simulink model "Assignment2_group4"  (R2020a)
settings: Solver=FixedStepAuto  StartTime=0.0  StopTime=10.0  FixedStep=1e-3  RelTol=1e-3  EnableMultiTasking=on
undefined symbols (not defined in the file): A0, A1, D0, D1, D10, D11, D12, D13, D2, D3, D4, D5, D6, D7, D8, D9, PTA0, PTA1, PTA2, PTB2, PTB23, PTB3, PTB9, PTC16, PTC17, PTC2, PTC3, PTC4, PTD0, PTD1, PTD2, PTD3
libraries: frdmk64flib x23, etargetslib x2
settings Model: ExtModeTrigDuration=5  Creator=win10  LastModifiedBy=win10
settings OptimizationCC: EnhancedBackFolding=on  PassReuseOutputArgsAs=Individual arguments  ZeroExternalMemoryAtStartup=off  ZeroInternalMemoryAtStartup=off  MaxStackSize=64  OptimizeBlockOrder=speed  DifferentSizesBufferReuse=on  OptimizationCustomize=off  EfficientTunableParamExpr=on
settings DebuggingCC: ParameterTunabilityLossMsg=error
settings HardwareCC: ProdBitPerPointer=32  ProdBitPerSizeT=32  ProdBitPerPtrDiffT=32  ProdLargestAtomicInteger=Long  ProdLargestAtomicFloat=Double  ProdWordSize=32  ProdHWDeviceType=ARM Compatible->ARM Cortex
settings SFSimCC: MATLABDynamicMemAlloc=off
settings RTWCC: SystemTargetFile=ert.tlc  HardwareBoard=NXP FRDM-K64F  TemplateMakefile=ert_default_tmf  Toolchain=GNU Tools for ARM Embedded Processors
settings CodeAppCC: ForceParamTrailComments=on  IgnoreCustomStorageClasses=off  OperatorAnnotations=on  SimulinkDataObjDesc=on  SFDataObjDesc=on  InsertBlockDesc=on

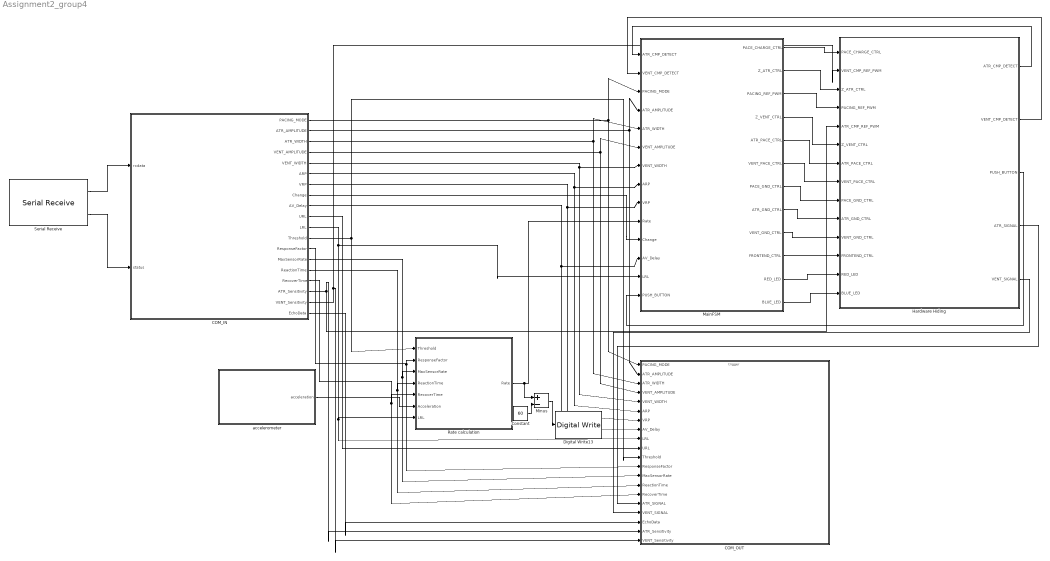
== system Assignment2_group4 ==
  COM_IN : Stateflow chart  TreatAsAtomicUnit=on
      settings: PortSchema="{\"entries\":[{\"content\":{\"sides\":[{\"content\":{\"connectorIds\":[\"In2\",\"In1\"]},\"type\":\"ConnectorPlacement.EquallySpacedRectSide\",\"uuid\":\"e3132103-f253-4432-b504-84705a150e61\"},{\"content\":{\"connectorIds\":[\"Out1\",\"Out2\",\"Out3\",\"Out4\",\"Out5\",\"Out6\",\"Out7\",\"Out8\",\"Out9\",\"Out10\",\"Out11\",\"Out12\",\"Out13\",\"Out14\",\"Out15\",\"Out16\",\"Out17\",\"Out18\",\"Out19\"],\"side\":\"RIGHT\"},\"type\":\"ConnectorPlacement.EquallySpacedRectSide\",\"uuid\":\"097bc9b8-1262-45b5-bb9b-69159a4df10c\"},{\"content\":{\"connectorIds\":[],\"side\":\"TOP\"},\"type\":\"ConnectorPlacement.EquallySpacedRectSide\",\"uuid\":\"fce19345-6d4b-4b3c-aee5-22ababb9e44d\"}]},\"type\":\"ConnectorPlacement.EquallySpacedConnector\",\"uuid\":\"5020afdc-7bbd-4924-8d59-6a0d5305ac11\"}],\"packageUris\":[\"http://schema.mathworks.com/mf0/Connector/19700101\"],\"version\":\"1.0\"}"
  COM_OUT : Subsystem  TreatAsAtomicUnit=on
  Constant : Constant  Value=60
  Digital Write13 : frdmk64flib/Digital Write  Whichpin=GREEN_LED
  Hardware Hiding : Subsystem
  MainFSM : Stateflow chart  TreatAsAtomicUnit=on
  Minus : Sum  Inputs=+-
  Rate calculation : Subsystem
  Serial Receive : frdmk64flib/Serial Receive  SCIModule=0  Baudrate=uint32(9600)  Parity=None  StopBits=1  HardwareFlowControl=None  ByteOrder=LittleEndian  DataType=uint8  DataLength=19  BlockingMode=off  OutputStatus=on  SampleTime=-1
  accelerometer : Subsystem
  wires:
  accelerometer/1(acceleration) -> Rate calculation/6(Acceleration)
  Rate calculation/1(Rate) -> Minus/1, MainFSM/10(Rate)
  Serial Receive/1 -> COM_IN/2(rxdata)
  Serial Receive/2 -> COM_IN/1(status)
  COM_IN/1(PACING_MODE) -> MainFSM/3(PACING_MODE), COM_OUT/1(PACING_MODE)
  COM_IN/5(VENT_WIDTH) -> COM_OUT/5(VENT_WIDTH), MainFSM/7(VENT_WIDTH)
  COM_IN/6(ARP) -> COM_OUT/6(ARP), MainFSM/8(ARP)
  COM_IN/7(VRP) -> COM_OUT/7(VRP), MainFSM/9(VRP)
  COM_IN/8(Change) -> MainFSM/11(Change)
  COM_IN/9(AV_Delay) -> COM_OUT/8(AV_Delay), MainFSM/12(AV_Delay)
  COM_IN/11(LRL) -> Rate calculation/7(LRL), COM_OUT/9(LRL), MainFSM/13(LRL)
  COM_IN/13(ResponseFactor) -> COM_OUT/12(ResponseFactor), Rate calculation/2(ResponseFactor)
  COM_IN/14(MaxSensorRate) -> COM_OUT/13(MaxSensorRate), Rate calculation/3(MaxSensorRate)
  COM_IN/15(ReactionTime) -> COM_OUT/14(ReactionTime), Rate calculation/4(ReactionTime)
  COM_IN/16(RecoverTime) -> Rate calculation/5(RecoverTime), COM_OUT/15(RecoverTime)
  COM_IN/10(URL) -> COM_OUT/10(URL)
  COM_IN/19(EchoData) -> COM_OUT/18(EchoData)
  COM_IN/3(ATR_WIDTH) -> MainFSM/5(ATR_WIDTH), COM_OUT/3(ATR_WIDTH)
  COM_IN/12(Threshold) -> COM_OUT/11(Threshold), Rate calculation/1(Threshold)
  COM_IN/4(VENT_AMPLITUDE) -> MainFSM/6(VENT_AMPLITUDE), COM_OUT/4(VENT_AMPLITUDE)
  COM_IN/2(ATR_AMPLITUDE) -> MainFSM/4(ATR_AMPLITUDE), COM_OUT/2(ATR_AMPLITUDE)
  COM_IN/17(ATR_Sensitivity) -> COM_OUT/19(ATR_Sensitivity), Hardware Hiding/5(ATR_CMP_REF_PWM)
  COM_IN/18(VENT_Sensitivity) -> Hardware Hiding/2(VENT_CMP_REF_PWM), COM_OUT/20(VENT_Sensitivity)
  MainFSM/1(PACE_CHARGE_CTRL) -> Hardware Hiding/1(PACE_CHARGE_CTRL)
  MainFSM/2(Z_ATR_CTRL) -> Hardware Hiding/3(Z_ATR_CTRL)
  MainFSM/3(PACING_REF_PWM) -> Hardware Hiding/4(PACING_REF_PWM)
  MainFSM/4(Z_VENT_CTRL) -> Hardware Hiding/6(Z_VENT_CTRL)
  MainFSM/5(ATR_PACE_CTRL) -> Hardware Hiding/7(ATR_PACE_CTRL)
  MainFSM/6(VENT_PACE_CTRL) -> Hardware Hiding/8(VENT_PACE_CTRL)
  MainFSM/7(PACE_GND_CTRL) -> Hardware Hiding/9(PACE_GND_CTRL)
  MainFSM/8(ATR_GND_CTRL) -> Hardware Hiding/10(ATR_GND_CTRL)
  MainFSM/9(VENT_GND_CTRL) -> Hardware Hiding/11(VENT_GND_CTRL)
  MainFSM/10(FRONTEND_CTRL) -> Hardware Hiding/12(FRONTEND_CTRL)
  MainFSM/11(RED_LED) -> Hardware Hiding/13(RED_LED)
  MainFSM/12(BLUE_LED) -> Hardware Hiding/14(BLUE_LED)
  Hardware Hiding/4(ATR_SIGNAL) -> COM_OUT/16(ATR_SIGNAL)
  Hardware Hiding/5(VENT_SIGNAL) -> COM_OUT/17(VENT_SIGNAL)
  Hardware Hiding/1(ATR_CMP_DETECT) -> MainFSM/1(ATR_CMP_DETECT)
  Hardware Hiding/2(VENT_CMP_DETECT) -> MainFSM/2(VENT_CMP_DETECT)
  Hardware Hiding/3(PUSH_BUTTON) -> MainFSM/14(PUSH_BUTTON)
  Constant/1 -> Minus/2
  Minus/1 -> Digital Write13/1

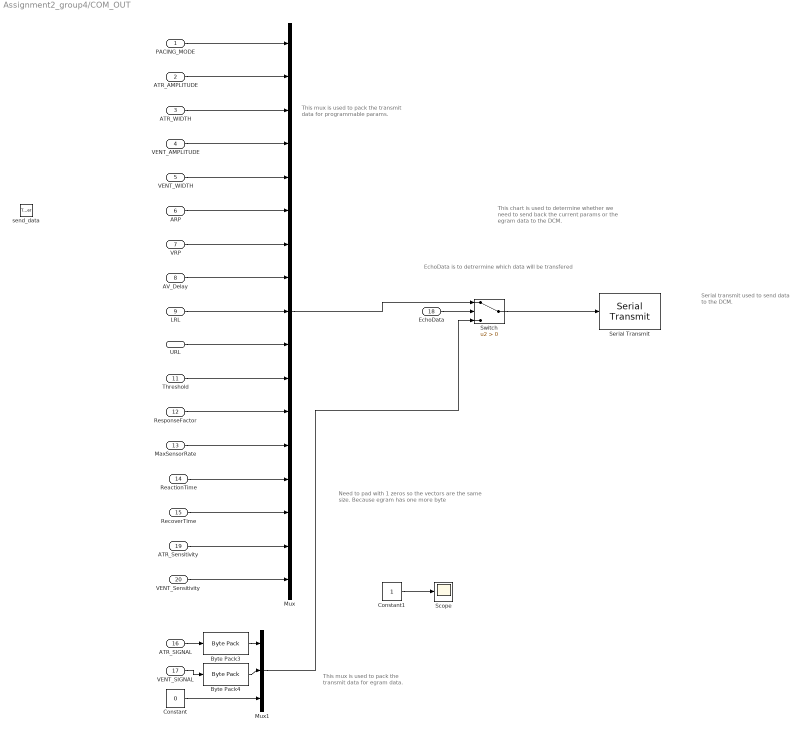
== system Assignment2_group4/COM_OUT ==
  note: EchoData is to detrermine which data will be transfered
  note: Serial transmit used to send data
      | to the DCM.
  note: This chart is used to determine whether
      | we need to send back the current params
      | or the egram data to the DCM.
  note: Need to pad with 1 zeros so the vectors
      | are the same size. Because egram has one more byte
  note: This mux is used to pack the
      | transmit data for egram data.
  note: This mux is used to pack the transmit
      | data for programmable params.
  PACING_MODE : Inport  OutDataTypeStr=uint8
  ATR_AMPLITUDE : Inport  Port=2  OutDataTypeStr=uint8
  ATR_WIDTH : Inport  Port=3  OutDataTypeStr=uint8
  VENT_AMPLITUDE : Inport  Port=4  OutDataTypeStr=uint8
  VENT_WIDTH : Inport  Port=5  OutDataTypeStr=uint8
  ARP : Inport  Port=6  OutDataTypeStr=uint8
  VRP : Inport  Port=7  OutDataTypeStr=uint8
  AV_Delay : Inport  Port=8  OutDataTypeStr=uint8
  LRL : Inport  Port=9  OutDataTypeStr=uint8
  URL : Inport  Port=10  OutDataTypeStr=uint8
  Threshold : Inport  Port=11  OutDataTypeStr=uint8
  ResponseFactor : Inport  Port=12  OutDataTypeStr=uint8
  MaxSensorRate : Inport  Port=13  OutDataTypeStr=uint8
  ReactionTime : Inport  Port=14  OutDataTypeStr=uint8
  RecoverTime : Inport  Port=15  OutDataTypeStr=uint8
  ATR_SIGNAL : Inport  Port=16  OutDataTypeStr=double
  VENT_SIGNAL : Inport  Port=17  OutDataTypeStr=double
  EchoData : Inport  Port=18
  ATR_Sensitivity : Inport  Port=19
  VENT_Sensitivity : Inport  Port=20
  send_data : TriggerPort  TriggerType=function-call  IsSimulinkFunction=on  FunctionName=send_data  VariantControl=Variant
  Byte Pack3 : etargetslib/Byte Pack  datatypes={'double'}  byteAlign=1
  Byte Pack4 : etargetslib/Byte Pack  datatypes={'double'}  byteAlign=1
  Constant : Constant  Value=0  OutDataTypeStr=uint8
  Constant1 : Constant
  Mux : Mux  Inputs=17
  Mux1 : Mux  Inputs=3
  Scope : Scope
  Serial Transmit : frdmk64flib/Serial Transmit  SCIModule=0  Baudrate=uint32(9600)  Parity=None  StopBits=1  HardwareFlowControl=None  ByteOrder=LittleEndian  BlockingMode=on  OutputStatus=off
  Switch : Switch  Criteria=u2 > Threshold
  wires:
  Switch/1 -> Serial Transmit/1
  ATR_AMPLITUDE/1 -> Mux/2
  ATR_WIDTH/1 -> Mux/3
  VENT_AMPLITUDE/1 -> Mux/4
  VENT_WIDTH/1 -> Mux/5
  ARP/1 -> Mux/6
  VRP/1 -> Mux/7
  AV_Delay/1 -> Mux/8
  LRL/1 -> Mux/9
  URL/1 -> Mux/10
  Threshold/1 -> Mux/11
  ResponseFactor/1 -> Mux/12
  MaxSensorRate/1 -> Mux/13
  ReactionTime/1 -> Mux/14
  RecoverTime/1 -> Mux/15
  Mux/1 -> Switch/1
  Mux1/1 -> Switch/3
  EchoData/1 -> Switch/2
  Byte Pack3/1 -> Mux1/1
  ATR_SIGNAL/1 -> Byte Pack3/1
  VENT_SIGNAL/1 -> Byte Pack4/1
  Byte Pack4/1 -> Mux1/2
  ATR_Sensitivity/1 -> Mux/16
  VENT_Sensitivity/1 -> Mux/17
  Constant/1 -> Mux1/3
  PACING_MODE/1 -> Mux/1
  Constant1/1 -> Scope/1

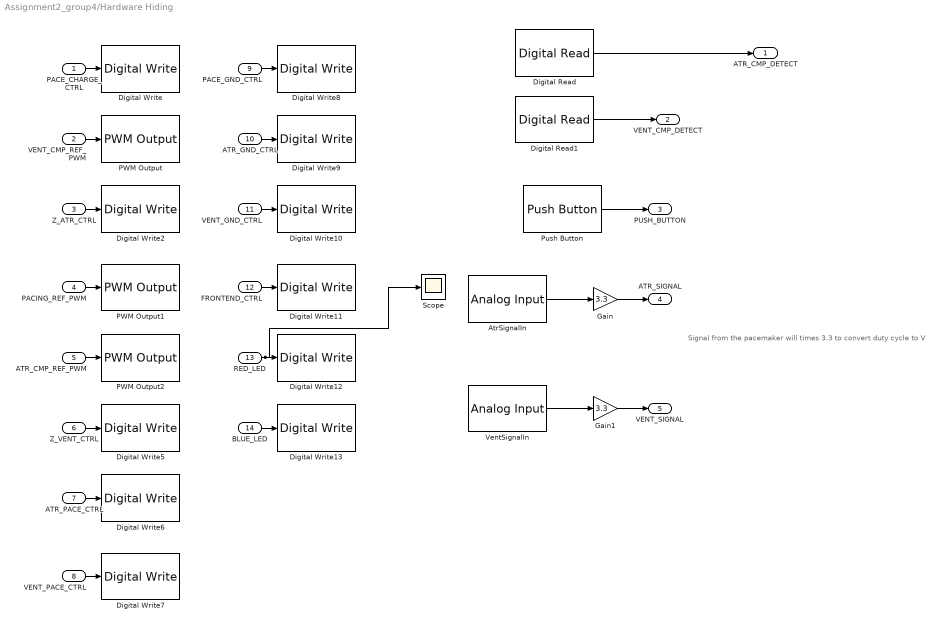
== system Assignment2_group4/Hardware Hiding ==
  note: Signal from the pacemaker will times 3.3 to convert duty cycle to V
  PACE_CHARGE_CTRL : Inport  OutDataTypeStr=boolean
  VENT_CMP_REF_PWM : Inport  Port=2  OutDataTypeStr=uint8
  Z_ATR_CTRL : Inport  Port=3  OutDataTypeStr=boolean
  PACING_REF_PWM : Inport  Port=4  OutDataTypeStr=uint8
  ATR_CMP_REF_PWM : Inport  Port=5  OutDataTypeStr=uint8
  Z_VENT_CTRL : Inport  Port=6  OutDataTypeStr=boolean
  ATR_PACE_CTRL : Inport  Port=7  OutDataTypeStr=boolean
  VENT_PACE_CTRL : Inport  Port=8  OutDataTypeStr=boolean
  PACE_GND_CTRL : Inport  Port=9  OutDataTypeStr=boolean
  ATR_GND_CTRL : Inport  Port=10  OutDataTypeStr=boolean
  VENT_GND_CTRL : Inport  Port=11  OutDataTypeStr=boolean
  FRONTEND_CTRL : Inport  Port=12  OutDataTypeStr=boolean
  RED_LED : Inport  Port=13  OutDataTypeStr=boolean
  BLUE_LED : Inport  Port=14  OutDataTypeStr=boolean
  AtrSignalIn : frdmk64flib/Analog Input  Whichpin=PTB2 (A0)  SampleTime=-1
  Digital Read : frdmk64flib/Digital Read  Whichpin=PTC16 (D0)  SampleTime=-1
  Digital Read1 : frdmk64flib/Digital Read  Whichpin=PTC17 (D1)  SampleTime=-1
  Digital Write : frdmk64flib/Digital Write  Whichpin=PTB9 (D2)
  Digital Write10 : frdmk64flib/Digital Write  Whichpin=PTD3 (D12)
  Digital Write11 : frdmk64flib/Digital Write  Whichpin=PTD1 (D13)
  Digital Write12 : frdmk64flib/Digital Write  Whichpin=RED_LED
  Digital Write13 : frdmk64flib/Digital Write  Whichpin=BLUE_LED
  Digital Write2 : frdmk64flib/Digital Write  Whichpin=PTB23 (D4)
  Digital Write5 : frdmk64flib/Digital Write  Whichpin=PTC3 (D7)
  Digital Write6 : frdmk64flib/Digital Write  Whichpin=PTA0 (D8)
  Digital Write7 : frdmk64flib/Digital Write  Whichpin=PTC4 (D9)
  Digital Write8 : frdmk64flib/Digital Write  Whichpin=PTD0 (D10)
  Digital Write9 : frdmk64flib/Digital Write  Whichpin=PTD2 (D11)
  Gain : Gain  Gain=3.3
  Gain1 : Gain  Gain=3.3
  PWM Output : frdmk64flib/PWM Output  Whichpin=PTA1 (D3)  InitialFrequency=2000  InitialDutyCycle=0
  PWM Output1 : frdmk64flib/PWM Output  Whichpin=PTA2 (D5)  InitialFrequency=2000  InitialDutyCycle=0
  PWM Output2 : frdmk64flib/PWM Output  Whichpin=PTC2 (D6)  InitialFrequency=2000  InitialDutyCycle=0
  Push Button : frdmk64flib/Push Button  Whichswitch=SW2  SampleTime1=-1
  Scope : Scope
  VentSignalIn : frdmk64flib/Analog Input  Whichpin=PTB3 (A1)  SampleTime=-1
  ATR_CMP_DETECT : Outport
  VENT_CMP_DETECT : Outport  Port=2
  PUSH_BUTTON : Outport  Port=3
  ATR_SIGNAL : Outport  Port=4
  VENT_SIGNAL : Outport  Port=5
  wires:
  PACE_CHARGE_CTRL/1 -> Digital Write/1
  VENT_CMP_REF_PWM/1 -> PWM Output/1
  PACING_REF_PWM/1 -> PWM Output1/1
  Z_ATR_CTRL/1 -> Digital Write2/1
  ATR_PACE_CTRL/1 -> Digital Write6/1
  VENT_PACE_CTRL/1 -> Digital Write7/1
  Z_VENT_CTRL/1 -> Digital Write5/1
  ATR_CMP_REF_PWM/1 -> PWM Output2/1
  BLUE_LED/1 -> Digital Write13/1
  VENT_GND_CTRL/1 -> Digital Write10/1
  FRONTEND_CTRL/1 -> Digital Write11/1
  ATR_GND_CTRL/1 -> Digital Write9/1
  PACE_GND_CTRL/1 -> Digital Write8/1
  Push Button/1 -> PUSH_BUTTON/1
  Digital Read1/1 -> VENT_CMP_DETECT/1
  VentSignalIn/1 -> Gain1/1
  Gain/1 -> ATR_SIGNAL/1
  Gain1/1 -> VENT_SIGNAL/1
  Digital Read/1 -> ATR_CMP_DETECT/1
  AtrSignalIn/1 -> Gain/1
  RED_LED/1 -> Scope/1, Digital Write12/1

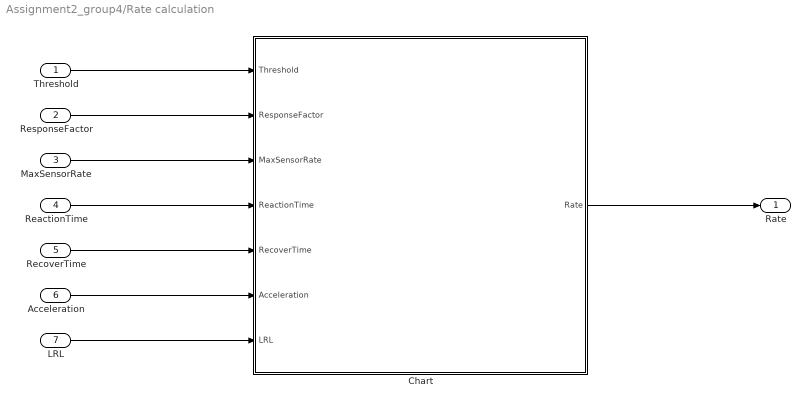
== system Assignment2_group4/Rate calculation ==
  Threshold : Inport  OutDataTypeStr=uint8
  ResponseFactor : Inport  Port=2  OutDataTypeStr=uint8
  MaxSensorRate : Inport  Port=3  OutDataTypeStr=uint8
  ReactionTime : Inport  Port=4  OutDataTypeStr=uint8
  RecoverTime : Inport  Port=5  OutDataTypeStr=uint8
  Acceleration : Inport  Port=6
  LRL : Inport  Port=7  OutDataTypeStr=uint8
  Chart : Stateflow chart  TreatAsAtomicUnit=on
  Rate : Outport
  wires:
  Threshold/1 -> Chart/1(Threshold)
  ResponseFactor/1 -> Chart/2(ResponseFactor)
  MaxSensorRate/1 -> Chart/3(MaxSensorRate)
  ReactionTime/1 -> Chart/4(ReactionTime)
  RecoverTime/1 -> Chart/5(RecoverTime)
  Acceleration/1 -> Chart/6(Acceleration)
  LRL/1 -> Chart/7(LRL)
  Chart/1(Rate) -> Rate/1

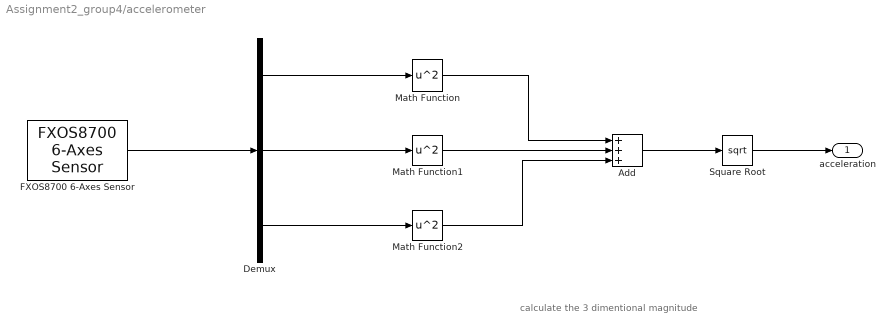
== system Assignment2_group4/accelerometer ==
  note: calculate the 3 dimentional magnitude
  Add : Sum  Inputs=+++
  Demux : Demux  Outputs=3
  FXOS8700 6-Axes Sensor : frdmk64flib/FXOS8700 6-Axes Sensor  Activesensor=Accelerometer only  ODR=800Hz  HybridODR=400Hz  Accelfullrange=-4g to +4g  SampleTime=0.01
  Math Function : Math  Operator=square  SaturateOnIntegerOverflow=on
  Math Function1 : Math  Operator=square  SaturateOnIntegerOverflow=on
  Math Function2 : Math  Operator=square  SaturateOnIntegerOverflow=on
  Square Root : Sqrt  SaturateOnIntegerOverflow=on
  acceleration : Outport
  wires:
  FXOS8700 6-Axes Sensor/1 -> Demux/1
  Demux/1 -> Math Function/1
  Demux/2 -> Math Function1/1
  Demux/3 -> Math Function2/1
  Math Function/1 -> Add/1
  Math Function1/1 -> Add/2
  Math Function2/1 -> Add/3
  Add/1 -> Square Root/1
  Square Root/1 -> acceleration/1

== stateflow chart Assignment2_group4/Rate calculation/Chart ==
  state Init
    entry:
    Rate = LRL;
  state Lower
    entry:
    NewRate = 0.8*ResponseFactor*(Acceleration-Threshold)+LRL;
    if NewRate >= MaxSensorRate
    NewRate = MaxSensorRate;
    end
    step = (NewRate-Rate)/ReactionTime;
  state Higher
    entry:
    step = (MaxSensorRate-LRL)/RecoverTime;
  state RateDecrease
    entry:
    Rate = Rate-step;
  state RateIncrease
    entry:
    Rate = Rate+step;
  (default) -> Init
  Higher -> Lower [order 1] : [Acceleration>=Threshold]
  Init -> Higher
  Lower -> Higher [order 1] : [Acceleration<Threshold]
  Higher -> RateDecrease [order 2] : after(200,msec)
  RateDecrease -> Higher
  RateIncrease -> Lower
  Lower -> RateIncrease [order 2] : after(200,msec)
  data: Threshold input uint8; ResponseFactor input uint8; MaxSensorRate input uint8; ReactionTime input uint8; RecoverTime input uint8; Acceleration input; LRL input uint8; Rate output; NewRate local; step local

== stateflow chart Assignment2_group4/COM_IN ==
  note: Unpacking the received serial data from the DCM
      | and setting the params to the values received.
  state SetParam
    entry:
    PACING_MODE = rxdata(3);
    ATR_AMPLITUDE = rxdata(4);
    VENT_AMPLITUDE = rxdata(5);
    ATR_WIDTH = rxdata(6);
    VENT_WIDTH = rxdata(7);
    AV_Delay = rxdata(8);
    ARP = rxdata(9);
    VRP = rxdata(10);
    Threshold = rxdata(11);
    LRL = rxdata(12);
    URL = rxdata(13);
    ReactionTime =rxdata(14);
    ResponseFactor = rxdata(15);
    RecoverTime = rxdata(16);
    MaxSensorRate = rxdata(17);
    ATR_Sensitivity = rxdata(18);
    VENT_Sensitivity = rxdata(19);
    Change = 1;
  note: Will initiate parameters when DCM
      | is not used
  state Init
    entry:
    PACING_MODE = 0;
    ATR_AMPLITUDE =75;
    VENT_AMPLITUDE = 75;
    ATR_WIDTH = 1;
    VENT_WIDTH = 1;
    AV_Delay = 150;
    ARP = 250;
    VRP = 250;
    Threshold = 50;
    LRL = 60;
    URL = 120;
    ReactionTime = 5;
    ResponseFactor = 10;
    RecoverTime = 5;
    MaxSensorRate = 120;
    ATR_Sensitivity = 8;
    VENT_Sensitivity = 8;
    Change = 0;
    %15+2 bytes total to be send
  state StandBy
  state EchoParam
    entry:
    EchoData = 1;
    send_data();
  state EchoEgram
    entry:
    EchoData = 0;
    send_data();
  note: calling send data function that transmit parameters back to the DCM
  note: calling send data function that transmit EGRAM back to the DCM
  (default) -> Init
  SetParam -> StandBy : after(2000,msec)
  (junction 37) -> SetParam [order 1] : [rxdata(2) == hex2dec('55')]
  Init -> StandBy
  StandBy -> (junction 37) : [status == 0 && rxdata(1) == hex2dec('16')]
  (junction 37) -> EchoEgram [order 3] : [after(2000,msec)&&rxdata(2) == hex2dec('47')]
  (junction 37) -> EchoParam [order 2] : [after(2000,msec)&&rxdata(2) == hex2dec('22')]
  EchoEgram -> StandBy : after(5000,msec)
  EchoParam -> StandBy : after(5000,msec)
  data: status input uint8; PACING_MODE output uint8; ATR_AMPLITUDE output uint8; ATR_WIDTH output uint8; VENT_AMPLITUDE output uint8; VENT_WIDTH output uint8; ARP output uint8; VRP output uint8; Change output uint8; AV_Delay output uint8; URL output uint8; LRL output uint8; Threshold output uint8; ResponseFactor output uint8; MaxSensorRate output uint8; ReactionTime output uint8; RecoverTime output uint8; ATR_Sensitivity output; VENT_Sensitivity output; EchoData output; rxdata input

== stateflow chart Assignment2_group4/MainFSM ==
  note: Transisition of DOO
  note: this is state is to charge the capacitor
      | by turn on the PACE_CHARGE_CTRL
      | and stop pacing a heart signal by turn on
      | the VENT_GND_CTRL and turn off the
      | VENT_PACE_CTRL
  note: this is state is to charge the capacitor
      | by turn on the PACE_CHARGE_CTRL
      | and stop pacing a heart signal by turn on
      | the ATR_GND_CTRL and turn off the
      | ATR_PACE_CTRL
  state V_Charging_VOO
    entry:
    PACE_CHARGE_CTRL = true;
    PACE_GND_CTRL = true;
    VENT_PACE_CTRL = false;
    Z_ATR_CTRL = false;
    Z_VENT_CTRL = false;
    ATR_PACE_CTRL = false;
    ATR_GND_CTRL = false;
    VENT_GND_CTRL = true;
    BLUE_LED = false;
    PACING_REF_PWM = VENT_AMPLITUDE;
  note: The state will move from charging the capacitor to discharging the capacitor
      | which is pacing a heart signal.
  state A_Charging_AOO
    entry:
    PACE_CHARGE_CTRL = true;
    PACE_GND_CTRL = true;
    VENT_PACE_CTRL = false;
    Z_ATR_CTRL = false;
    Z_VENT_CTRL = false;
    ATR_PACE_CTRL = false;
    ATR_GND_CTRL = true;
    VENT_GND_CTRL = false;
    RED_LED = false;
    PACING_REF_PWM = ATR_AMPLITUDE;
  note: PACING_MODE:
      | 0:AOO
      | 1:VOO
      | 2:AAI
      | 3:VVI
      | 4:DOO
      | 5:AOOR
      | 6:VOOR
      | 7:AAIR
      | 8:VVIR
      | 9:DOOR
  state V_Pacing
    entry:
    PACE_CHARGE_CTRL = false;
    PACE_GND_CTRL = true;
    ATR_PACE_CTRL = false;
    ATR_GND_CTRL = false;
    VENT_PACE_CTRL = true;
    VENT_GND_CTRL = false;
    Z_ATR_CTRL = false;
    Z_VENT_CTRL = false;
    BLUE_LED = true;
  state V_Charging_VVI
    entry:
    PACE_CHARGE_CTRL = true;
    PACE_GND_CTRL = true;
    VENT_PACE_CTRL = false;
    Z_ATR_CTRL = false;
    Z_VENT_CTRL = false;
    ATR_PACE_CTRL = false;
    ATR_GND_CTRL = false;
    VENT_GND_CTRL = true;
    BLUE_LED = false;
    PACING_REF_PWM = VENT_AMPLITUDE;
  state A_pacing
    entry:
    PACE_CHARGE_CTRL = false;
    PACE_GND_CTRL = true;
    ATR_PACE_CTRL = true;
    ATR_GND_CTRL = false;
    VENT_PACE_CTRL = false;
    VENT_GND_CTRL = false;
    Z_ATR_CTRL = false;
    Z_VENT_CTRL = false;
    RED_LED = true;
  state A_Charging_AAI
    entry:
    FRONTEND_CTRL = true;
    PACE_CHARGE_CTRL = true;
    PACE_GND_CTRL = true;
    VENT_PACE_CTRL = false;
    Z_ATR_CTRL = false;
    Z_VENT_CTRL = false;
    ATR_PACE_CTRL = false;
    ATR_GND_CTRL = true;
    VENT_GND_CTRL = false;
    RED_LED = false;
    PACING_REF_PWM = ATR_AMPLITUDE;
  note: This state will move the current from C22 capacitor to perform signal
      | by turn off PACE_CHARGE_CTRL and turn on PACE_END_CTRL
      | and turn on VENT_PACE_CTRL to pace in the vent
  note: This state will move the current from C22 capacitor to perform signal
      | by turn off PACE_CHARGE_CTRL and turn on PACE_END_CTRL
      | and turn on ATR_PACE_CTRL to pace in the atrium
  note: This initial state, all switch are open circuit and no current to charge the capacitor as well as pacing
      | FRONTEND_CTRL is on to sense the circuitry  and will output heart signal based on whcih pacing mode
  note: This loop state is for sensing mode. The sensing mode will begin after ARP delay and
      | will process if ATR_CMP_DETECT is higher than threshold to prevent next pacing
      | signal. The pushbutton is to perform a natural heart signal to inhibit next pacing signal
  note: This loop state is for sensing mode. The sensing mode will begin after VRP delay and
      | will process if VENT_CMP_DETECT is higher than threshold to prevent next pacing
      | signal. The pushbutton is to perform a natural heart signal to inhibit next pacing signal
  state Init
    entry:
    FRONTEND_CTRL = true;
    PACE_CHARGE_CTRL = false;
    ATR_PACE_CTRL = false;
    VENT_PACE_CTRL = false;
    ATR_GND_CTRL = false;
    VENT_GND_CTRL = false;
    PACE_GND_CTRL = false;
    PACING_REF_PWM = 0;
    BLUE_LED = false;
    RED_LED = false;
  state V_Charging_VOOR
    entry:
    PACE_CHARGE_CTRL = true;
    PACE_GND_CTRL = true;
    VENT_PACE_CTRL = false;
    Z_ATR_CTRL = false;
    Z_VENT_CTRL = false;
    ATR_PACE_CTRL = false;
    ATR_GND_CTRL = false;
    VENT_GND_CTRL = true;
    BLUE_LED = false;
    PACING_REF_PWM = VENT_AMPLITUDE;
  state A_Charging_AOOR
    entry:
    PACE_CHARGE_CTRL = true;
    PACE_GND_CTRL = true;
    VENT_PACE_CTRL = false;
    Z_ATR_CTRL = false;
    Z_VENT_CTRL = false;
    ATR_PACE_CTRL = false;
    ATR_GND_CTRL = true;
    VENT_GND_CTRL = false;
    RED_LED = false;
    PACING_REF_PWM = ATR_AMPLITUDE;
  state V_Charging_VViR
    entry:
    PACE_CHARGE_CTRL = true;
    PACE_GND_CTRL = true;
    VENT_PACE_CTRL = false;
    Z_ATR_CTRL = false;
    Z_VENT_CTRL = false;
    ATR_PACE_CTRL = false;
    ATR_GND_CTRL = false;
    VENT_GND_CTRL = true;
    BLUE_LED = false;
    PACING_REF_PWM = VENT_AMPLITUDE;
  state A_Charging_AAIR
    entry:
    PACE_CHARGE_CTRL = true;
    PACE_GND_CTRL = true;
    VENT_PACE_CTRL = false;
    Z_ATR_CTRL = false;
    Z_VENT_CTRL = false;
    ATR_PACE_CTRL = false;
    ATR_GND_CTRL = true;
    VENT_GND_CTRL = false;
    RED_LED = false;
    PACING_REF_PWM = ATR_AMPLITUDE;
  note: Transition of DOOR
  V_Pacing -> A_Charging_AOO [order 4] : [after(VENT_WIDTH,msec)&&PACING_MODE==4]
  A_pacing -> V_Charging_VOO [order 4] : [after(ATR_WIDTH,msec)&&PACING_MODE==4]
  V_Charging_VOO -> V_Pacing [order 2] : [after(60000/uint16(LRL)-uint16(VENT_WIDTH),msec)&&PACING_MODE==1]
  Init -> V_Charging_VOO [order 8] : [PACING_MODE==1]
  A_Charging_AOO -> A_pacing [order 1] : [after(60/uint16(LRL)*1000-uint16(ATR_WIDTH),msec)&&PACING_MODE==0]
  V_Pacing -> V_Charging_VOO [order 1] : [after(VENT_WIDTH,msec)&&PACING_MODE==1]
  A_pacing -> A_Charging_AOO [order 3] : [after(ATR_WIDTH,msec)&&PACING_MODE==0]
  V_Charging_VOO -> Init [order 1] : [Change == 1]
  Init -> A_Charging_AOO [order 1] : [PACING_MODE==0 || PACING_MODE==4]
  A_Charging_AOO -> Init [order 2] : [Change ==1]
  V_Charging_VOO -> V_Pacing [order 3] : [after(AV_Delay-ATR_WIDTH,msec)&&PACING_MODE==4]
  A_Charging_AOO -> A_pacing [order 3] : [after(60/uint16(LRL)*1000-uint16(VENT_WIDTH)-uint16(AV_Delay),msec)&&PACING_MODE==4]
  Init -> V_Charging_VVI [order 4] : [PACING_MODE==3]
  V_Charging_VVI -> V_Pacing [order 1] : after(60/uint16(LRL)*1000-uint16(VENT_WIDTH)-uint16(VRP),msec)
  A_Charging_AAI -> A_pacing [order 1] : after(60/uint16(LRL)*1000-uint16(ATR_WIDTH)-uint16(ARP),msec)
  Init -> A_Charging_AAI [order 2] : [PACING_MODE==2]
  V_Charging_VVI -> Init [order 3] : [Change==1]
  V_Charging_VViR -> V_Pacing [order 2] : [after(60/uint16(Rate)*1000-uint16(VENT_WIDTH)-uint16(VRP),msec)]
  V_Pacing -> V_Charging_VVI [order 2] : [after(VENT_WIDTH,msec)&&PACING_MODE==3]
  A_Charging_AAI -> Init [order 3] : [Change==1]
  A_pacing -> A_Charging_AAI [order 1] : [after(ATR_WIDTH,msec)&&PACING_MODE==2]
  A_pacing -> A_Charging_AAIR [order 5] : [after(ATR_WIDTH,msec)&&PACING_MODE==7]
  V_Pacing -> V_Charging_VViR [order 5] : [after(VENT_WIDTH,msec)&&PACING_MODE==8]
  A_Charging_AAIR -> A_pacing [order 2] : after(60/uint16(Rate)*1000-uint16(ATR_WIDTH)-uint16(ARP),msec)
  V_Charging_VVI -> V_Charging_VVI [order 2] : [[after(VRP,msec) && VENT_CMP_DETECT == false || PUSH_BUTTON ==true]]
  V_Pacing -> A_Charging_AOOR [order 6] : [after(VENT_WIDTH,msec)&&PACING_MODE==9]
  V_Charging_VOOR -> V_Pacing [order 1] : [after(60/uint16(Rate)*1000-uint16(VENT_WIDTH),msec)&&PACING_MODE==6]
  V_Pacing -> V_Charging_VOOR [order 3] : [after(VENT_WIDTH,msec)&&PACING_MODE==6]
  V_Charging_VOOR -> V_Pacing [order 3] : [after(AV_Delay-ATR_WIDTH,msec)&&PACING_MODE==9]
  (default) -> Init
  A_Charging_AAI -> A_Charging_AAI [order 2] : [after(ARP,msec)&&ATR_CMP_DETECT== true || PUSH_BUTTON ==true]
  A_pacing -> V_Charging_VOOR [order 6] : [after(ATR_WIDTH,msec)&&PACING_MODE==9]
  A_Charging_AOOR -> A_pacing [order 2] : [after(60/uint16(Rate)*1000-uint16(ATR_WIDTH),msec)&&PACING_MODE==5]
  A_pacing -> A_Charging_AOOR [order 2] : [after(ATR_WIDTH,msec)&&PACING_MODE==5]
  A_Charging_AOOR -> A_pacing [order 3] : [after(60/uint16(Rate)*1000-uint16(VENT_WIDTH)-uint16(AV_Delay),msec)&&PACING_MODE==9]
  Init -> A_Charging_AOOR [order 3] : [PACING_MODE ==5 || PACING_MODE==9]
  Init -> V_Charging_VOOR [order 5] : [PACING_MODE==6]
  A_Charging_AOOR -> Init [order 1] : [Change == 1]
  V_Charging_VOOR -> Init [order 2] : [Change==1]
  V_Charging_VViR -> Init [order 1] : [Change==1]
  Init -> V_Charging_VViR [order 7] : [PACING_MODE==8]
  A_Charging_AAIR -> Init [order 1] : [Change==1]
  Init -> A_Charging_AAIR [order 6] : [PACING_MODE==7 ]
  V_Charging_VViR -> V_Charging_VViR [order 3] : [[after(VRP,msec) && VENT_CMP_DETECT == true || PUSH_BUTTON ==true]]
  A_Charging_AAIR -> A_Charging_AAIR [order 3] : [after(ARP,msec) && ATR_CMP_DETECT == true || PUSH_BUTTON ==true]
  data: ATR_CMP_DETECT input; VENT_CMP_DETECT input; PACING_MODE input uint8; ATR_AMPLITUDE input uint8; ATR_WIDTH input uint8; VENT_AMPLITUDE input uint8; VENT_WIDTH input uint8; ARP input uint8; VRP input uint8; Rate input; Change input uint8; AV_Delay input uint8; LRL input uint8; PUSH_BUTTON input boolean; PACE_CHARGE_CTRL output boolean; Z_ATR_CTRL output boolean; PACING_REF_PWM output uint8; Z_VENT_CTRL output boolean; ATR_PACE_CTRL output boolean; VENT_PACE_CTRL output boolean; PACE_GND_CTRL output boolean; ATR_GND_CTRL output boolean; VENT_GND_CTRL output boolean; FRONTEND_CTRL output boolean; RED_LED output boolean; BLUE_LED output boolean
